simulink model "Hinf_2DOFsimulation"  (R2023a)
settings: Solver=VariableStepAuto  StartTime=0.0  StopTime=100  RelTol=1e-3
values from neighbouring files (symbols this model uses):
  C = [1 0 0 0; 0 1 0 0]    [Hinf_1DOF.m]    (also in Hinf_2DOFinit.m; Hinf_U_init.m; Hinf_WU_init.m; Hinf_init.m)
  dtheta_0 = 0    [Hinf_1DOF.m]    (also in Hinf_2DOFinit.m; Hinf_U_init.m; Hinf_WU_init.m; Hinf_init.m)
  dz_0 = 0    [Hinf_1DOF.m]    (also in Hinf_2DOFinit.m; Hinf_U_init.m; Hinf_WU_init.m; Hinf_init.m)
  fa_w = 0    [Hinf_1DOF.m]    (also in Hinf_2DOFinit.m; Hinf_U_init.m; Hinf_WU_init.m; Hinf_init.m)
  fm_w = s_param.g*s_param.m    [Hinf_1DOF.m]    (also in Hinf_2DOFinit.m; Hinf_U_init.m; Hinf_WU_init.m; Hinf_init.m)
  K = tf(ss(K.A,K.B,K.C,K.D))    [Hinf_U_init.m]    (also in Hinf_WU_init.m; Hinf_init.m)
  K_fsf = -place(A,B,[-0.01 -0.01 -0.5 -0.5])    [Hinf_2DOFinit.m]
  Km1 = 1.1    [Hinf_1DOF.m]    (also in Hinf_2DOFinit.m; Hinf_U_init.m; Hinf_WU_init.m; Hinf_init.m)
  Km2 = 1.1    [Hinf_1DOF.m]    (also in Hinf_2DOFinit.m; Hinf_U_init.m; Hinf_WU_init.m; Hinf_init.m)
  out_rate = 0.001    [Hinf_1DOF.m]    (also in Hinf_2DOFinit.m; Hinf_U_init.m; Hinf_WU_init.m; Hinf_init.m)
  T1 = 0.05    [Hinf_1DOF.m]    (also in Hinf_2DOFinit.m; Hinf_U_init.m; Hinf_WU_init.m; Hinf_init.m)
  T2 = 0.15    [Hinf_1DOF.m]    (also in Hinf_2DOFinit.m; Hinf_U_init.m; Hinf_WU_init.m; Hinf_init.m)
  theta_0_real = theta_0 + std_dev.theta_0*randn(1,1)    [Hinf_1DOF.m]    (also in Hinf_2DOFinit.m = theta_0+std_dev.theta_0*randn(1,1); Hinf_U_init.m = theta_0+std_dev.theta_0*randn(1,1); Hinf_WU_init.m = theta_0+std_dev.theta_0*randn(1,1); Hinf_init.m = theta_0+std_dev.theta_0*randn(1,1))
  theta_w = 0    [Hinf_1DOF.m]    (also in Hinf_2DOFinit.m; Hinf_U_init.m; Hinf_WU_init.m; Hinf_init.m)
  Tm1 = 1    [Hinf_1DOF.m]    (also in Hinf_2DOFinit.m; Hinf_U_init.m; Hinf_WU_init.m; Hinf_init.m)
  Tm2 = 1    [Hinf_1DOF.m]    (also in Hinf_2DOFinit.m; Hinf_U_init.m; Hinf_WU_init.m; Hinf_init.m)
  x_0 = [z_0; theta_0; dz_0; dtheta_0]    [Hinf_1DOF.m]    (also in Hinf_2DOFinit.m; Hinf_U_init.m; Hinf_WU_init.m; Hinf_init.m)
  z_0_real = z_0 + std_dev.z_0*randn(1,1)    [Hinf_1DOF.m]    (also in Hinf_2DOFinit.m = z_0+std_dev.z_0*randn(1,1); Hinf_U_init.m = z_0+std_dev.z_0*randn(1,1); Hinf_WU_init.m = z_0+std_dev.z_0*randn(1,1); Hinf_init.m = z_0+std_dev.z_0*randn(1,1))
  z_w = 200    [Hinf_1DOF.m]    (also in Hinf_2DOFinit.m = 400; Hinf_U_init.m = 400; Hinf_WU_init.m = 400; Hinf_init.m = 400)
undefined symbols (not defined in the file or in its folder): std_dev
libraries: simulink x2
settings Model: Creator=franc  LastModifiedBy=franc

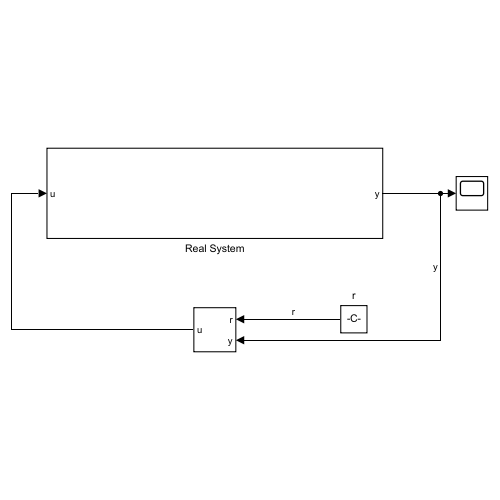
[thumbnail: Simulink's stored preview of the top-level diagram]
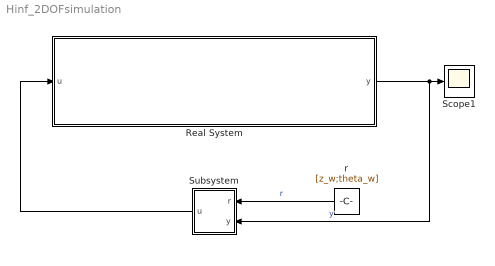
== system Hinf_2DOFsimulation ==
  Real System : Subsystem
  Scope1 : Scope
  Subsystem : Subsystem
  r : Constant  Value=[z_w;theta_w]
  wires:
  Real System/1(y) -> Scope1/1, Subsystem/2(y)  "y"
  r/1 -> Subsystem/1(r)  "r"
  Subsystem/1(u) -> Real System/1(u)

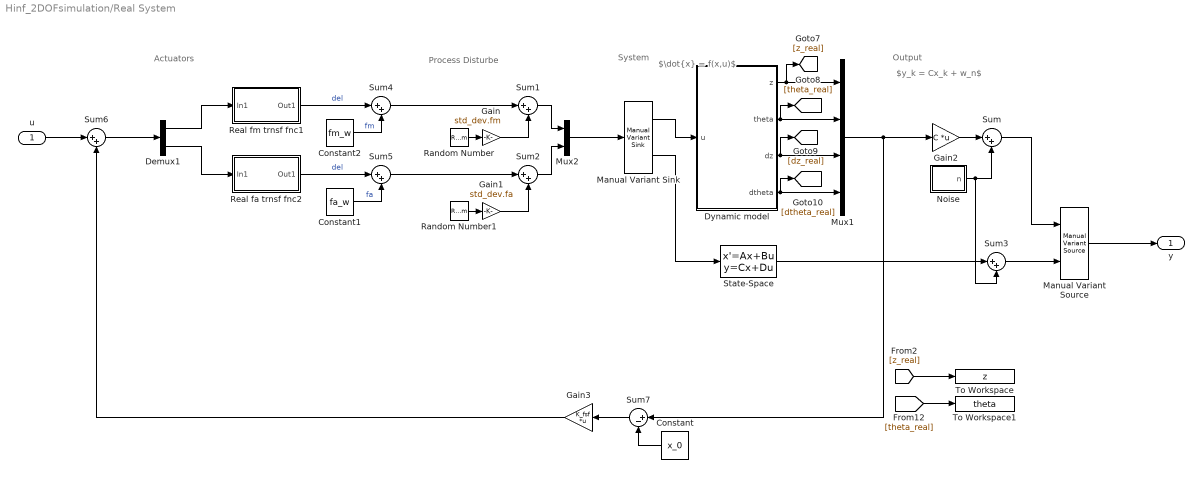
== system Hinf_2DOFsimulation/Real System ==
  note: Process Disturbe
  note: System
  note: $y_k = Cx_k + w_n$
  note: $\dot{x} = f(x,u)$
  note: Output
  note: Actuators
  u : Inport
  Constant : Constant  Value=x_0
  Constant1 : Constant  Value=fa_w
  Constant2 : Constant  Value=fm_w
  Demux1 : Demux  Outputs=2
  Dynamic model : Subsystem
  Gain : Gain  Gain=std_dev.fm
  Gain1 : Gain  Gain=std_dev.fa
  Gain2 : Gain  Gain=C  Multiplication=Matrix(K*u)
  Gain3 : Gain  Gain=K_fsf  Multiplication=Matrix(K*u)
  Manual Variant Sink : simulink/Signal Routing/Manual Variant Sink  NumChoices=2  LabelModeActiveChoice=V_1
  Manual Variant Source : simulink/Signal Routing/Manual Variant Source  NumChoices=2  LabelModeActiveChoice=V_1
  Mux1 : Mux
  Mux2 : Mux  Inputs=2
  Noise : Subsystem
  Random Number : RandomNumber  SampleTime=out_rate
  Random Number1 : RandomNumber  SampleTime=out_rate
  Real fa trnsf fnc2 : Subsystem
  Real fm trnsf fnc1 : Subsystem
  State-Space : StateSpace  InitialCondition=0
  Sum{,1..6} (7 alike) : Sum  Inputs=|++
  Sum7 : Sum  Inputs=|+-
  To Workspace : ToWorkspace  VariableName=z  SaveFormat=Timeseries  SampleTime=-1
  To Workspace1 : ToWorkspace  VariableName=theta  SaveFormat=Timeseries  SampleTime=-1
  y : Outport
  wires:
  Manual Variant Sink/1 -> Dynamic model/1(u)
  Constant2/1 -> Sum4/2  "fm"
  Demux1/1 -> Real fm trnsf fnc1/1(In1)
  Real fm trnsf fnc1/1(Out1) -> Sum4/1  "del"
  Sum2/1 -> Mux2/2
  Dynamic model/4(dtheta) -> Mux1/4, [dtheta_real]
  Mux2/1 -> Manual Variant Sink/1
  Gain2/1 -> Sum/1
  Dynamic model/2(theta) -> Mux1/2, [theta_real]
  Sum5/1 -> Sum2/1
  Dynamic model/3(dz) -> Mux1/3, [dz_real]
  Noise/1(n) -> Sum/2, Sum3/2
  Demux1/2 -> Real fa trnsf fnc2/1(In1)
  Dynamic model/1(z) -> [z_real], Mux1/1
  Sum3/1 -> Manual Variant Source/2
  Gain1/1 -> Sum2/2
  Sum1/1 -> Mux2/1
  u/1 -> Sum6/1
  State-Space/1 -> Sum3/1
  Mux1/1 -> Sum7/1, Gain2/1
  Sum/1 -> Manual Variant Source/1
  Sum4/1 -> Sum1/1
  Constant1/1 -> Sum5/2  "fa"
  Real fa trnsf fnc2/1(Out1) -> Sum5/1  "del"
  Manual Variant Sink/2 -> State-Space/1
  Gain/1 -> Sum1/2
  Random Number/1 -> Gain/1
  Random Number1/1 -> Gain1/1
  Manual Variant Source/1 -> y/1
  [z_real] -> To Workspace/1
  [theta_real] -> To Workspace1/1
  Sum6/1 -> Demux1/1
  Sum7/1 -> Gain3/1
  Constant/1 -> Sum7/2
  Gain3/1 -> Sum6/2

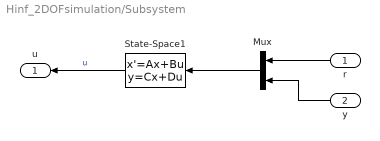
== system Hinf_2DOFsimulation/Subsystem ==
  r : Inport
  y : Inport  Port=2
  Mux : Mux  Inputs=2
  State-Space1 : StateSpace  A=K.A  B=K.B  C=K.C  D=K.D  InitialCondition=0
  u : Outport
  wires:
  r/1 -> Mux/1
  Mux/1 -> State-Space1/1
  y/1 -> Mux/2
  State-Space1/1 -> u/1  "u"

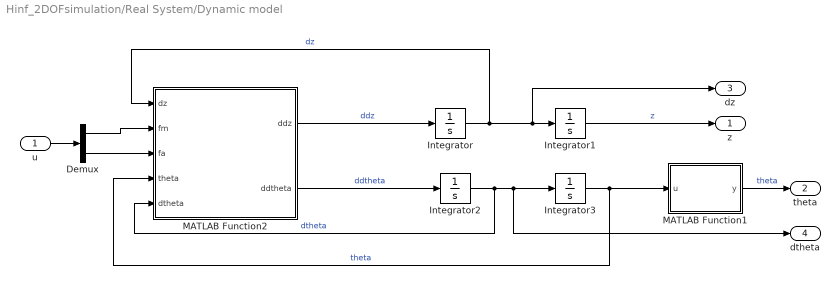
== system Hinf_2DOFsimulation/Real System/Dynamic model ==
  u : Inport
  Demux : Demux  Outputs=2
  Integrator : Integrator  InitialCondition=dz_0
  Integrator1 : Integrator  InitialCondition=z_0_real
  Integrator2 : Integrator  InitialCondition=dtheta_0
  Integrator3 : Integrator  InitialCondition=theta_0_real
  MATLAB Function1 : MATLAB Function  TreatAsAtomicUnit=on
  MATLAB Function2 : MATLAB Function  TreatAsAtomicUnit=on
  z : Outport
  theta : Outport  Port=2
  dz : Outport  Port=3
  dtheta : Outport  Port=4
  wires:
  Integrator3/1 -> MATLAB Function2/4(theta), MATLAB Function1/1(u)  "theta"
  Integrator2/1 -> dtheta/1, Integrator3/1, MATLAB Function2/5(dtheta)  "dtheta"
  MATLAB Function1/1(y) -> theta/1  "theta"
  Integrator1/1 -> z/1  "z"
  MATLAB Function2/2(ddtheta) -> Integrator2/1  "ddtheta"
  MATLAB Function2/1(ddz) -> Integrator/1  "ddz"
  Integrator/1 -> dz/1, Integrator1/1, MATLAB Function2/1(dz)  "dz"
  u/1 -> Demux/1
  Demux/2 -> MATLAB Function2/3(fa)
  Demux/1 -> MATLAB Function2/2(fm)

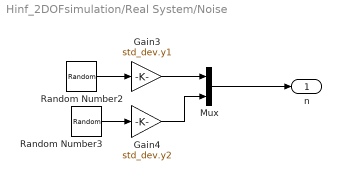
== system Hinf_2DOFsimulation/Real System/Noise ==
  Gain3 : Gain  Gain=std_dev.y1
  Gain4 : Gain  Gain=std_dev.y2
  Mux : Mux  Inputs=2
  Random Number2 : RandomNumber  SampleTime=0.1
  Random Number3 : RandomNumber  SampleTime=0.1
  n : Outport
  wires:
  Random Number2/1 -> Gain3/1
  Random Number3/1 -> Gain4/1
  Gain4/1 -> Mux/2
  Mux/1 -> n/1
  Gain3/1 -> Mux/1

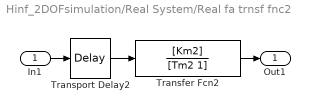
== system Hinf_2DOFsimulation/Real System/Real fa trnsf fnc2 ==
  In1 : Inport
  Transfer Fcn2 : TransferFcn  Numerator=[Km2]  Denominator=[Tm2 1]
  Transport Delay2 : TransportDelay  DelayTime=T2
  Out1 : Outport
  wires:
  Transport Delay2/1 -> Transfer Fcn2/1
  Transfer Fcn2/1 -> Out1/1
  In1/1 -> Transport Delay2/1

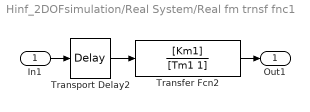
== system Hinf_2DOFsimulation/Real System/Real fm trnsf fnc1 ==
  In1 : Inport
  Transfer Fcn2 : TransferFcn  Numerator=[Km1]  Denominator=[Tm1 1]
  Transport Delay2 : TransportDelay  DelayTime=T1
  Out1 : Outport
  wires:
  In1/1 -> Transport Delay2/1
  Transfer Fcn2/1 -> Out1/1
  Transport Delay2/1 -> Transfer Fcn2/1

== matlab function Hinf_2DOFsimulation/Real System/Dynamic model/MATLAB Function2 ==
  data: dz input; fm input; fa input; ddz output; ddtheta output; theta input; dtheta input; s_param parameter
function [ddz, ddtheta] = fcn(dz, fm, fa, theta, dtheta, s_param)

% Rename params
J = s_param.J;     
m = s_param.m;     
b = s_param.b;      
beta = s_param.beta;    
g = s_param.g;     
l = s_param.l;   

%% Dynamic equations

ddz = -b/m * dz + fm/m * cos(theta) -g;
ddtheta = -beta/J * dtheta + 2 * l/J * fa;

end

== matlab function Hinf_2DOFsimulation/Real System/Dynamic model/MATLAB Function1 ==
  data: u input; y output
function y = fcn(u)

y = atan2(sin(u), cos(u));
end
